simulink model "Subsystem"  (R2020a)
settings: Solver=ode45  StartTime=0.0  StopTime=0.2  RelTol=1e-3
model workspace (MAT data in the model file):
  K = 0.0274
values from neighbouring files (symbols this model uses):
  b = 3.5077E-6    [motor.sldd]    (also in pos.mat = 3.5077e-06)
  J = 3.2284E-6    [motor.sldd]    (also in pos.mat = 3.2284e-06)
  L = 2.75e-06    [pos.mat]
  R = 4.0    [motor.sldd]    (also in pos.mat = 4)
settings Model: DataDictionary=motor.sldd  Creator=sansh  LastModifiedBy=Admin
settings DataIOCC: SaveOutput=off  SaveTime=off  ReturnWorkspaceOutputs=off
settings DebuggingCC: ArithmeticOperatorsInVariantConditions=warning
settings SFSimCC: SimUseLocalCustomCode=off  CustomCodeUndefinedFunction=UseInterfaceOnly
settings RTWCC: RTWUseLocalCustomCode=off
settings CodeAppCC: StateflowObjectComments=on

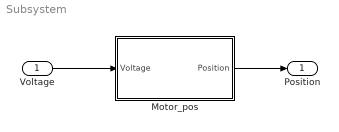
== system Subsystem ==
  Voltage : Inport  OutDataTypeStr=double  PortDimensions=1  SampleTime=0
  Motor_pos : Subsystem
  Position : Outport  OutDataTypeStr=double  PortDimensions=1  SampleTime=0
  wires:
  Motor_pos/1(Position) -> Position/1
  Voltage/1 -> Motor_pos/1(Voltage)

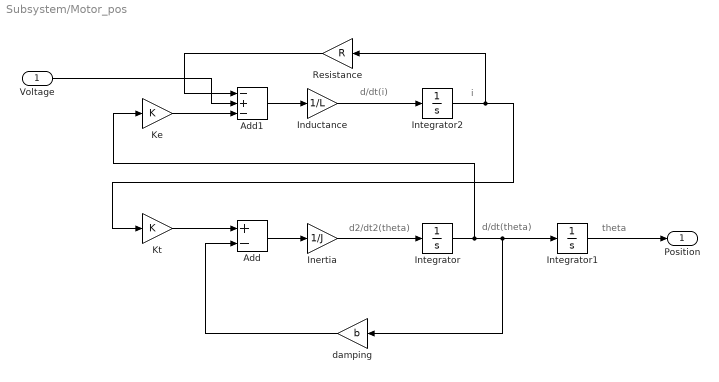
== system Subsystem/Motor_pos ==
  note: theta
  note: d/dt(theta)
  note: d2/dt2(theta)
  note: d/dt(i)
  note: i
  Voltage : Inport
  Add : Sum  Inputs=+-
  Add1 : Sum  Inputs=-+-
  Inductance : Gain  Gain=1/L
  Inertia : Gain  Gain=1/J
  Integrator : Integrator
  Integrator1 : Integrator
  Integrator2 : Integrator
  Ke : Gain  Gain=K
  Kt : Gain  Gain=K
  Resistance : Gain  Gain=R
  damping : Gain  Gain=b
  Position : Outport
  wires:
  Add1/1 -> Inductance/1
  Ke/1 -> Add1/3
  Resistance/1 -> Add1/1
  Kt/1 -> Add/1
  damping/1 -> Add/2
  Add/1 -> Inertia/1
  Voltage/1 -> Add1/2
  Integrator1/1 -> Position/1
  Integrator/1 -> Integrator1/1, damping/1, Ke/1
  Integrator2/1 -> Kt/1, Resistance/1
  Inductance/1 -> Integrator2/1
  Inertia/1 -> Integrator/1
